simulink model "satball"  (R2023a)
settings: Solver=FixedStepDiscrete  StartTime=0.0  StopTime=inf  FixedStep=0.1  RelTol=1e-3  EnableMultiTasking=on
PreLoadFcn:
  | setenv('ROS_MASTER_URI','http://localhost:11311/');
  | setenv('ROS_IP','localhost');
  | rosinit('http://localhost:11311/',...
  |     'NodeHost','localhost',...
  |     'NodeName','/simulink_teststand');
undefined symbols (not defined in the file or in its folder): Quaternion
libraries: aausat3_lib x9, robotlib x4, simulink_need_slupdate x1
CloseFcn:
  | rosshutdown
settings Model: Creator=jn  LastModifiedBy=jacobel-omar
settings SolverCC: AlgebraicLoopSolver=TrustRegion
settings DataIOCC: SaveFormat=Array  ReturnWorkspaceOutputs=off
settings OptimizationCC: BlockReduction=off  DefaultParameterBehavior=Inlined  BufferReuse=off  ZeroExternalMemoryAtStartup=off  ZeroInternalMemoryAtStartup=off  LifeSpan=Inf  MaxStackSize=64  EfficientTunableParamExpr=on
settings DebuggingCC: SolverPrmCheckMsg=warning  UnconnectedInputMsg=warning  UnconnectedOutputMsg=warning  UnconnectedLineMsg=warning  AllowSymbolicDim=off  SFUnexpectedBacktrackingDiag=warning  SFNoUnconditionalDefaultTransitionDiag=warning  SFExecutionAtInitializationDiag=none  ArithmeticOperatorsInVariantConditions=warning
settings HardwareCC: ProdBitPerInt=16  ProdBitPerPointer=16  ProdBitPerSizeT=16  ProdBitPerPtrDiffT=16  ProdLargestAtomicFloat=None  ProdWordSize=16  ProdHWDeviceType=Atmel->AVR (8-bit)
settings ModelReferenceCC: EnableRefExpFcnMdlSchedulingChecks=on  PropagateSignalLabelsOutOfModel=off
settings SFSimCC: SimUseLocalCustomCode=off  MATLABDynamicMemAlloc=off  CustomCodeUndefinedFunction=UseInterfaceOnly  SimTargetLang=C++
settings RTWCC: Description=Embedded Coder  SystemTargetFile=ert.tlc  HardwareBoard=Robot Operating System (ROS)  TemplateMakefile=ert_default_tmf  GenerateReport=on  RTWUseLocalCustomCode=off  Toolchain=Catkin  IncludeHyperlinkInReport=on  LaunchReport=on  TargetLang=C++  GenerateTraceInfo=on  GenerateTraceReport=on  GenerateTraceReportSl=on  GenerateTraceReportSf=on  GenerateTraceReportEml=on
settings CodeAppCC: ForceParamTrailComments=on  OperatorAnnotations=on  SimulinkDataObjDesc=on  SFDataObjDesc=on  MATLABFcnDesc=on  InsertBlockDesc=on  StateflowObjectComments=on  MATLABSourceComments=on
settings ERTTargetCC: MultiwordLength=2048  CodeInterfacePackaging=C++ class  RootIOFormat=Structure reference
settings ConfigComp: CovMetricSettings=dw  CovSaveCumulativeToWorkspaceVar=on  CovSaveSingleToWorkspaceVar=on  CovExternalEMLEnable=off  CovSFcnEnable=off

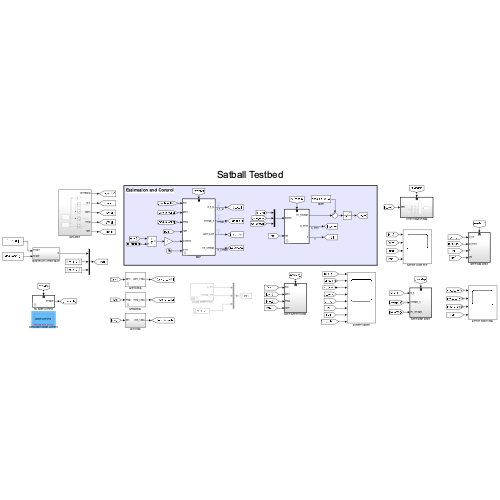
[thumbnail: Simulink's stored preview of the top-level diagram]
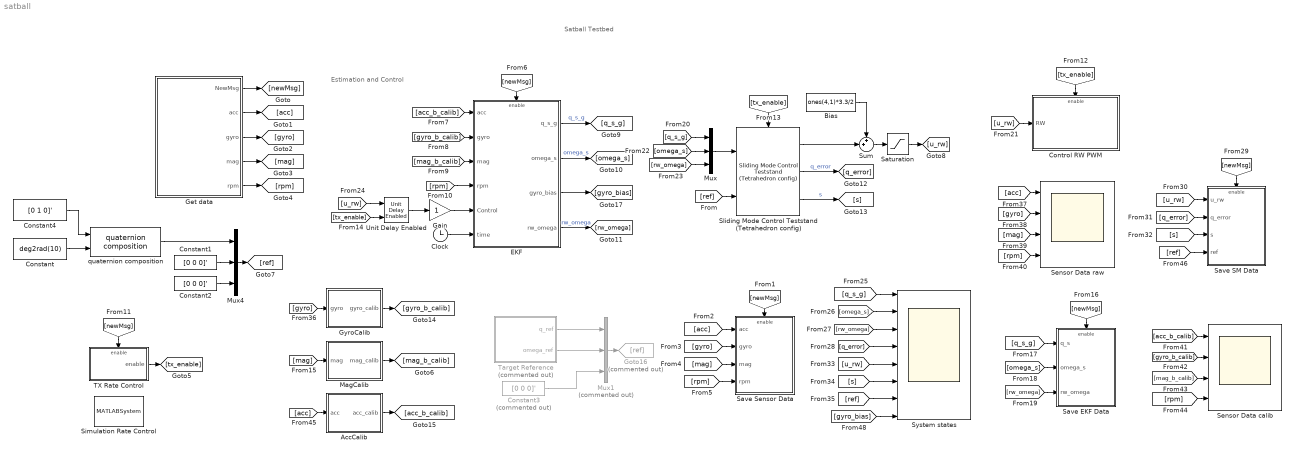
== system satball ==
  note: Estimation and Control
  note: Satball Testbed
  AccCalib : Subsystem
  Bias : Constant  Value=ones(4,1)*3.3/2
  Clock : Clock
  Constant : Constant  Value=deg2rad(10)
  Constant1 : Constant  Value=[0 0 0]'
  Constant2 : Constant  Value=[0 0 0]'
  Constant3 : Constant  Commented=on  Value=[0 0 0]'
  Constant4 : Constant  Value=[0 1 0]'
  Control RW PWM : Subsystem
  EKF : Subsystem  mask{Ts=-1, x0=[[0 0 0 1] [0 0 0] [3.443e-2 10.0104e-3 2.586e-3] [800 800 800 800]]', q_s_c=[0 0 0 1]', q_s_th=[0 0 1 0]'}
      mask prompts: Ts "Sampling time [s]"; x0 "Initial state vector"; q_s_c "Rotation from body to Control frame"; q_s_th "Rotation from body to Tetrahedron"
  Gain : Gain
  Get data : Subsystem
  Goto16 : Goto  Commented=on  GotoTag=ref
  GyroCalib : Subsystem  mask{bias=[0  0   0]', K_gyro=1.3316e-04}
      mask prompts: K_gyro "Sensor gain"
  MagCalib : Subsystem  mask{bias=|, U=|, q_g_mag=[0 0 0 1]', q_mag_b=[0 0 0 1]'}
      mask bias=|
      | [-8.8193
      |   130.0580
      |   202.0582]'
      mask U=|
      | [0.6339   -0.0215    0.0031;
      |          0    0.5742    0.0418;
      |          0         0    0.5785]*1.0e-03
      mask prompts: U "Calibration ellipsoide  matrix"; q_g_mag "Rotation from Global reference frame to local magnetic vector field"; q_mag_b "Magnetometer rotation to satellite body"
  Mux : Mux  Inputs=3
  Mux1 : Mux  Commented=on  Inputs=3
  Mux4 : Mux  Inputs=3
  Saturation : Saturate  UpperLimit=4  LowerLimit=0.1
  Save EKF Data : Subsystem
  Save SM Data : Subsystem
  Save Sensor Data : Subsystem
  Sensor Data calib : Scope  NumInputPorts=4
  Sensor Data raw : Scope  NumInputPorts=4
  Simulation Rate Control : MATLABSystem  System=ExampleHelperSimulationRateControl  SampleTime=0.1
      mask Type: ExampleHelperSimulationRateControl
      mask Display: disp('Rate Control');
  Sliding Mode Control Teststand (Tetrahedron config) : aausat3_lib/ACS/Sliding Mode Control Teststand (Tetrahedron config)  K=diag([1 1 1])*5  delta_0=3  e=90e-5  q_s_c=[0 0 0 1]'  q_s_tetra=[0 0 1 0]'  max_disturbance=6.0306e-04  enable_coriolis=on  Ts=1  Js=[0.6714 0.7044 0.7268]*1e-3  Jrw=[0.4513 0.4513 0.3811]*1e-6  Vcc=3.3
      settings: SourceProductName=AAUSAT3
  Sum : Sum  Inputs=++|
  System states : Scope  NumInputPorts=8
  TX Rate Control : Subsystem  mask{ts=10}
      mask prompts: ts "Number of Ticks to wait"
  Target Reference : Subsystem  Commented=on  mask{t_init=60, slope=0.1, offset=1.4}
      mask prompts: t_init "Time offset"; slope "maximum slope"; offset "angular offset"
  Unit Delay Enabled : simulink_need_slupdate/Unit Delay Enabled  vinit=0.0  tsamp=-1
  quaternion composition : aausat3_lib/Math Utilities/Quaternion operations/quaternion composition  SystemSampleTime=-1  VariantActivationTime=update diagram  Latency=0  AutoFrameSizeCalculation=off
      settings: SourceProductName=AAUSAT3
  wires:
  Get data/1(NewMsg) -> [newMsg]
  Get data/2(acc) -> [acc]
  Get data/3(gyro) -> [gyro]
  Get data/4(mag) -> [mag]
  Get data/5(rpm) -> [rpm]
  [newMsg] -> Save Sensor Data/Enable
  [acc] -> Save Sensor Data/1(acc)
  [gyro] -> Save Sensor Data/2(gyro)
  [mag] -> Save Sensor Data/3(mag)
  [rpm] -> Save Sensor Data/4(rpm)
  [newMsg] -> EKF/Enable
  [acc_b_calib] -> EKF/1(acc)
  [gyro_b_calib] -> EKF/2(gyro)
  [rpm] -> EKF/4(rpm)
  [newMsg] -> TX Rate Control/Enable
  [tx_enable] -> Control RW PWM/Enable
  TX Rate Control/1(enable) -> [tx_enable]
  Sliding Mode Control Teststand (Tetrahedron config)/2 -> [q_error]  "q_error"
  Sliding Mode Control Teststand (Tetrahedron config)/3 -> [s]  "s"
  [ref] -> Sliding Mode Control Teststand (Tetrahedron config)/2
  Mux/1 -> Sliding Mode Control Teststand (Tetrahedron config)/1
  Mux4/1 -> [ref]
  quaternion composition/1 -> Mux4/1
  Constant1/1 -> Mux4/2
  Constant2/1 -> Mux4/3
  [tx_enable] -> Sliding Mode Control Teststand (Tetrahedron config)/Enable
  Sliding Mode Control Teststand (Tetrahedron config)/1 -> Sum/2
  Bias/1 -> Sum/1
  Sum/1 -> Saturation/1
  [u_rw] -> Control RW PWM/1(RW)
  [tx_enable] -> Unit Delay Enabled/2
  [mag] -> MagCalib/1(mag)
  [mag_b_calib] -> EKF/3(mag)
  [newMsg] -> Save EKF Data/Enable
  [q_s_g] -> Save EKF Data/1(q_s)
  [omega_s] -> Save EKF Data/2(omega_s)
  [rw_omega] -> Save EKF Data/3(rw_omega)
  Saturation/1 -> [u_rw]
  EKF/1(q_s_g) -> [q_s_g]  "q_s_g"
  EKF/4(rw_omega) -> [rw_omega]  "rw_omega"
  EKF/2(omega_s) -> [omega_s]  "omega_s"
  [q_s_g] -> Mux/1
  [omega_s] -> Mux/2
  [rw_omega] -> Mux/3
  [u_rw] -> Unit Delay Enabled/1
  [q_s_g] -> System states/1
  [omega_s] -> System states/2
  [rw_omega] -> System states/3
  [q_error] -> System states/4
  [newMsg] -> Save SM Data/Enable
  [u_rw] -> Save SM Data/1(u_rw)
  [q_error] -> Save SM Data/2(q_error)
  [s] -> Save SM Data/3(s)
  [u_rw] -> System states/5
  [s] -> System states/6
  [ref] -> System states/7
  MagCalib/1(mag_calib) -> [mag_b_calib]
  Unit Delay Enabled/1 -> Gain/1
  [gyro] -> GyroCalib/1(gyro)
  GyroCalib/1(gyro_calib) -> [gyro_b_calib]
  [acc] -> Sensor Data raw/1
  [gyro] -> Sensor Data raw/2
  [mag] -> Sensor Data raw/3
  [rpm] -> Sensor Data raw/4
  [acc_b_calib] -> Sensor Data calib/1
  [gyro_b_calib] -> Sensor Data calib/2
  [mag_b_calib] -> Sensor Data calib/3
  [rpm] -> Sensor Data calib/4
  [acc] -> AccCalib/1(acc)
  AccCalib/1(acc_calib) -> [acc_b_calib]
  Gain/1 -> EKF/5(Control)
  Mux1/1 -> Goto16/1
  Target Reference/1(q_ref) -> Mux1/1
  Target Reference/2(omega_ref) -> Mux1/2
  Constant3/1 -> Mux1/3
  [ref] -> Save SM Data/4(ref)
  Constant/1 -> quaternion composition/2
  Constant4/1 -> quaternion composition/1
  Clock/1 -> EKF/6(time)
  EKF/3(gyro_bias) -> [gyro_bias]
  [gyro_bias] -> System states/8

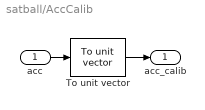
== system satball/AccCalib ==
  acc : Inport
  To unit vector : aausat3_lib/Math Utilities/Vector operations/To unit vector  SystemSampleTime=-1  VariantActivationTime=update diagram  Latency=0  AutoFrameSizeCalculation=off
      settings: SourceProductName=AAUSAT3
  acc_calib : Outport
  wires:
  acc/1 -> To unit vector/1
  To unit vector/1 -> acc_calib/1

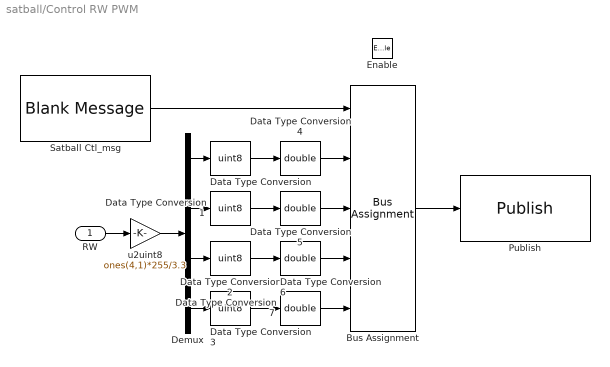
== system satball/Control RW PWM ==
  RW : Inport
  Enable : EnablePort
  Bus Assignment : BusAssignment  AssignedSignals=Quaternion.X,Quaternion.Y,Quaternion.Z,Quaternion.W
  Data Type Conversion{,1..3} (4 alike) : DataTypeConversion  OutDataTypeStr=uint8  RndMeth=Floor
  Data Type Conversion{4..7} (4 alike) : DataTypeConversion  OutDataTypeStr=double  RndMeth=Floor
  Demux : Demux
  Publish : robotlib/Publish  topicSource=Select from ROS network  topic=/satball/ctl  messageType=geometry_msgs/QuaternionStamped  legacyBusStruct=off  messageQueueLength=1
  Satball Ctl_msg : robotlib/Blank Message  messageClass=Message  entityType=geometry_msgs/QuaternionStamped  messageType=geometry_msgs/QuaternionStamped  SampleTime=-1  legacyBusStruct=off
  u2uint8 : Gain  Gain=ones(4,1)*255/3.3
  wires:
  Bus Assignment/1 -> Publish/1
  Satball Ctl_msg/1 -> Bus Assignment/1
  Demux/4 -> Data Type Conversion3/1
  Demux/3 -> Data Type Conversion2/1
  Demux/2 -> Data Type Conversion1/1
  Demux/1 -> Data Type Conversion/1
  Data Type Conversion/1 -> Data Type Conversion4/1
  Data Type Conversion1/1 -> Data Type Conversion5/1
  Data Type Conversion2/1 -> Data Type Conversion6/1
  Data Type Conversion3/1 -> Data Type Conversion7/1
  RW/1 -> u2uint8/1
  Data Type Conversion4/1 -> Bus Assignment/2
  Data Type Conversion5/1 -> Bus Assignment/3
  Data Type Conversion6/1 -> Bus Assignment/4
  Data Type Conversion7/1 -> Bus Assignment/5
  u2uint8/1 -> Demux/1

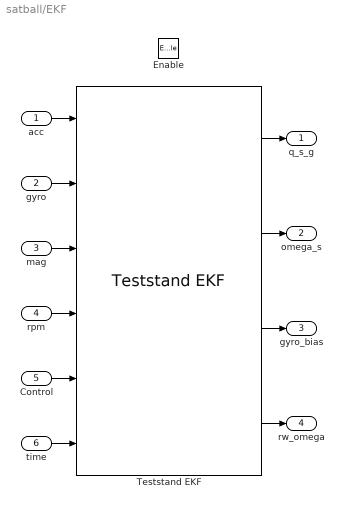
== system satball/EKF ==
  acc : Inport
  gyro : Inport  Port=2
  mag : Inport  Port=3
  rpm : Inport  Port=4
  Control : Inport  Port=5
  time : Inport  Port=6
  Enable : EnablePort
  Teststand EKF : aausat3_lib/ADS/Teststand EKF  dt=Ts  x0=x0  q_s_c=q_s_c  q_s_tetra=q_s_th
      settings: SourceProductName=AAUSAT3
  q_s_g : Outport
  omega_s : Outport  Port=2
  gyro_bias : Outport  Port=3
  rw_omega : Outport  Port=4
  wires:
  acc/1 -> Teststand EKF/1
  mag/1 -> Teststand EKF/3
  rpm/1 -> Teststand EKF/4
  gyro/1 -> Teststand EKF/2
  Teststand EKF/3 -> gyro_bias/1
  Teststand EKF/2 -> omega_s/1
  Teststand EKF/1 -> q_s_g/1
  Control/1 -> Teststand EKF/5
  time/1 -> Teststand EKF/6
  Teststand EKF/4 -> rw_omega/1

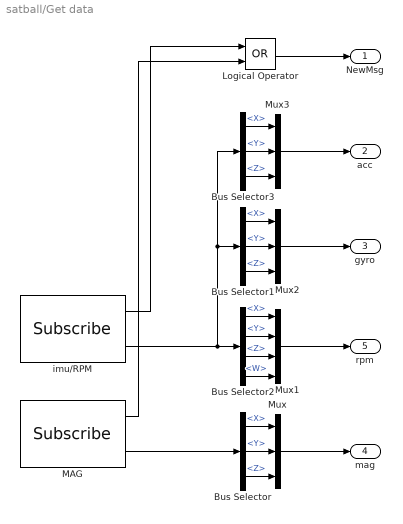
== system satball/Get data ==
  Bus Selector : BusSelector  OutputSignals=MagneticField_.X,MagneticField_.Y,MagneticField_.Z
  Bus Selector1 : BusSelector  OutputSignals=AngularVelocity.X,AngularVelocity.Y,AngularVelocity.Z
  Bus Selector2 : BusSelector  OutputSignals=Orientation.X,Orientation.Y,Orientation.Z,Orientation.W
  Bus Selector3 : BusSelector  OutputSignals=LinearAcceleration.X,LinearAcceleration.Y,LinearAcceleration.Z
  Logical Operator : Logic  Operator=OR  AllPortsSameDT=off  OutDataTypeStr=boolean
  MAG : robotlib/Subscribe  topicSource=Select from ROS network  topic=/satball/mag  messageType=sensor_msgs/MagneticField  SampleTime=-1  legacyBusStruct=off  messageQueueLength=1
  Mux : Mux  Inputs=3
  Mux1 : Mux
  Mux2 : Mux  Inputs=3
  Mux3 : Mux  Inputs=3
  imu/RPM : robotlib/Subscribe  topicSource=Select from ROS network  topic=/satball/imu_rpm  messageType=sensor_msgs/Imu  SampleTime=-1  legacyBusStruct=off  messageQueueLength=1
  NewMsg : Outport
  acc : Outport  Port=2
  gyro : Outport  Port=3
  mag : Outport  Port=4
  rpm : Outport  Port=5
  wires:
  MAG/1 -> Logical Operator/2
  imu/RPM/1 -> Logical Operator/1
  MAG/2 -> Bus Selector/1
  Bus Selector/2 -> Mux/2  "<Y>"
  Bus Selector/1 -> Mux/1  "<X>"
  Bus Selector/3 -> Mux/3  "<Z>"
  Mux/1 -> mag/1
  Logical Operator/1 -> NewMsg/1
  Bus Selector2/2 -> Mux1/2  "<Y>"
  Bus Selector2/1 -> Mux1/1  "<X>"
  Bus Selector2/3 -> Mux1/3  "<Z>"
  Mux1/1 -> rpm/1
  Bus Selector1/2 -> Mux2/2  "<Y>"
  Bus Selector1/1 -> Mux2/1  "<X>"
  Bus Selector1/3 -> Mux2/3  "<Z>"
  Bus Selector3/2 -> Mux3/2  "<Y>"
  Bus Selector3/1 -> Mux3/1  "<X>"
  Bus Selector3/3 -> Mux3/3  "<Z>"
  imu/RPM/2 -> Bus Selector3/1, Bus Selector1/1, Bus Selector2/1
  Bus Selector2/4 -> Mux1/4  "<W>"
  Mux3/1 -> acc/1
  Mux2/1 -> gyro/1

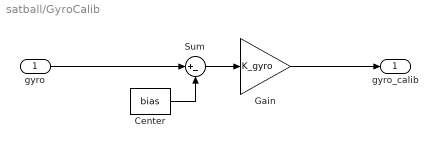
== system satball/GyroCalib ==
  gyro : Inport
  Center : Constant  Value=bias
  Gain : Gain  Gain=K_gyro
  Sum : Sum  Inputs=|+-
  gyro_calib : Outport
  wires:
  Center/1 -> Sum/2
  gyro/1 -> Sum/1
  Gain/1 -> gyro_calib/1
  Sum/1 -> Gain/1

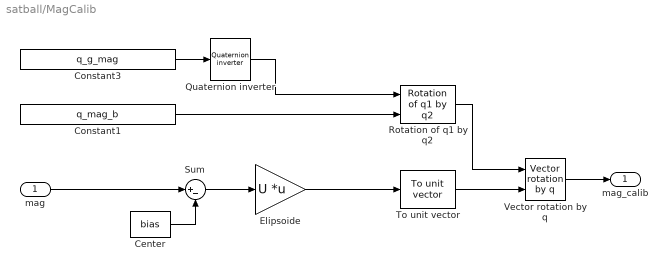
== system satball/MagCalib ==
  mag : Inport
  Center : Constant  Value=bias
  Constant1 : Constant  Value=q_mag_b
  Constant3 : Constant  Value=q_g_mag
  Elipsoide : Gain  Gain=U  Multiplication=Matrix(K*u) (u vector)
  Quaternion inverter : aausat3_lib/Math Utilities/Quaternion operations/Quaternion inverter  SystemSampleTime=-1  VariantActivationTime=update diagram  Latency=0  AutoFrameSizeCalculation=off
      settings: SourceProductName=AAUSAT3
  Rotation of q1 by q2 : aausat3_lib/Math Utilities/Quaternion operations/Rotation of q1 by q2  SystemSampleTime=-1  VariantActivationTime=update diagram  Latency=0  AutoFrameSizeCalculation=off
      settings: SourceProductName=AAUSAT3
  Sum : Sum  Inputs=|+-
  To unit vector : aausat3_lib/Math Utilities/Vector operations/To unit vector  SystemSampleTime=-1  VariantActivationTime=update diagram  Latency=0  AutoFrameSizeCalculation=off
      settings: SourceProductName=AAUSAT3
  Vector rotation by q : aausat3_lib/Math Utilities/Quaternion operations/Vector rotation by q  SystemSampleTime=-1  VariantActivationTime=update diagram  Latency=0  AutoFrameSizeCalculation=off
      settings: SourceProductName=AAUSAT3
  mag_calib : Outport
  wires:
  Center/1 -> Sum/2
  Sum/1 -> Elipsoide/1
  Constant3/1 -> Quaternion inverter/1
  Elipsoide/1 -> To unit vector/1
  Rotation of q1 by q2/1 -> Vector rotation by q/1
  Quaternion inverter/1 -> Rotation of q1 by q2/1
  Constant1/1 -> Rotation of q1 by q2/2
  To unit vector/1 -> Vector rotation by q/2
  Vector rotation by q/1 -> mag_calib/1
  mag/1 -> Sum/1

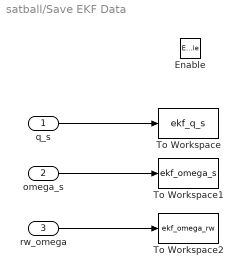
== system satball/Save EKF Data ==
  q_s : Inport
  omega_s : Inport  Port=2
  rw_omega : Inport  Port=3
  Enable : EnablePort
  To Workspace : ToWorkspace  VariableName=ekf_q_s  SaveFormat=Timeseries  SampleTime=-1
  To Workspace1 : ToWorkspace  VariableName=ekf_omega_s  SaveFormat=Timeseries  SampleTime=-1
  To Workspace2 : ToWorkspace  VariableName=ekf_omega_rw  SaveFormat=Timeseries  SampleTime=-1
  wires:
  q_s/1 -> To Workspace/1
  omega_s/1 -> To Workspace1/1
  rw_omega/1 -> To Workspace2/1

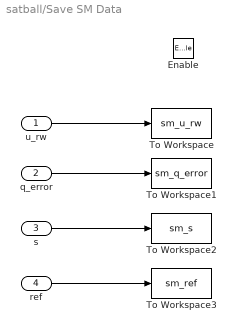
== system satball/Save SM Data ==
  u_rw : Inport
  q_error : Inport  Port=2
  s : Inport  Port=3
  ref : Inport  Port=4
  Enable : EnablePort
  To Workspace : ToWorkspace  VariableName=sm_u_rw  SaveFormat=Timeseries  SampleTime=-1
  To Workspace1 : ToWorkspace  VariableName=sm_q_error  SaveFormat=Timeseries  SampleTime=-1
  To Workspace2 : ToWorkspace  VariableName=sm_s  SaveFormat=Timeseries  SampleTime=-1
  To Workspace3 : ToWorkspace  VariableName=sm_ref  SaveFormat=Timeseries  SampleTime=-1
  wires:
  u_rw/1 -> To Workspace/1
  q_error/1 -> To Workspace1/1
  s/1 -> To Workspace2/1
  ref/1 -> To Workspace3/1

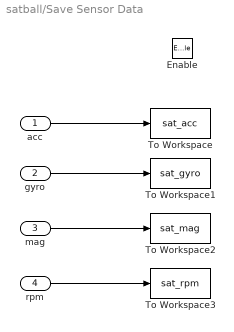
== system satball/Save Sensor Data ==
  acc : Inport
  gyro : Inport  Port=2
  mag : Inport  Port=3
  rpm : Inport  Port=4
  Enable : EnablePort
  To Workspace : ToWorkspace  VariableName=sat_acc  SaveFormat=Timeseries  SampleTime=-1
  To Workspace1 : ToWorkspace  VariableName=sat_gyro  SaveFormat=Timeseries  SampleTime=-1
  To Workspace2 : ToWorkspace  VariableName=sat_mag  SaveFormat=Timeseries  SampleTime=-1
  To Workspace3 : ToWorkspace  VariableName=sat_rpm  SaveFormat=Timeseries  SampleTime=-1
  wires:
  acc/1 -> To Workspace/1
  gyro/1 -> To Workspace1/1
  rpm/1 -> To Workspace3/1
  mag/1 -> To Workspace2/1

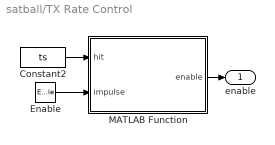
== system satball/TX Rate Control ==
  Enable : EnablePort  ShowOutputPort=on
  Constant2 : Constant  Value=ts
  MATLAB Function : MATLAB Function  TreatAsAtomicUnit=on
  enable : Outport  OutDataTypeStr=boolean
  wires:
  Constant2/1 -> MATLAB Function/1(hit)
  Enable/1 -> MATLAB Function/2(impulse)
  MATLAB Function/1(enable) -> enable/1

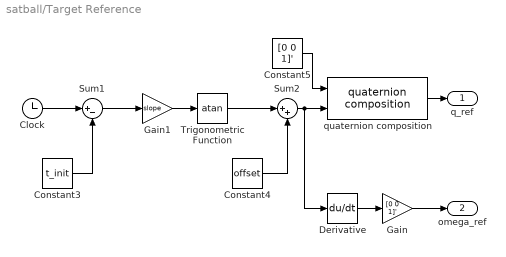
== system satball/Target Reference ==
  Clock : Clock
  Constant3 : Constant  Value=t_init
  Constant4 : Constant  Value=offset
  Constant5 : Constant  Value=[0 0 1]'
  Derivative : Derivative
  Gain : Gain  Gain=[0 0 1]'
  Gain1 : Gain  Gain=slope
  Sum1 : Sum  Inputs=|+-
  Sum2 : Sum  Inputs=|++
  Trigonometric Function : Trigonometry  Operator=atan
  quaternion composition : aausat3_lib/Math Utilities/Quaternion operations/quaternion composition
      settings: SourceProductName=AAUSAT3
  q_ref : Outport
  omega_ref : Outport  Port=2
  wires:
  Constant5/1 -> quaternion composition/1
  Constant3/1 -> Sum1/2
  Clock/1 -> Sum1/1
  Trigonometric Function/1 -> Sum2/1
  quaternion composition/1 -> q_ref/1
  Sum1/1 -> Gain1/1
  Sum2/1 -> Derivative/1, quaternion composition/2
  Constant4/1 -> Sum2/2
  Gain1/1 -> Trigonometric Function/1
  Gain/1 -> omega_ref/1
  Derivative/1 -> Gain/1

== matlab function satball/TX Rate Control/MATLAB Function ==
  data: hit input; enable output; impulse input
function enable = tx_enable(hit,impulse)

enable = tx_counter(hit,impulse);
